simulink model "DP_STD_MDL_Boost"  (R2025a)
settings: Solver=VariableStepAuto  StartTime=0.0  StopTime=1  RelTol=1e-3
libraries: spsSeriesRLCBranchLib x4, peripheral_utilities x3, spsMosfetLib x2, spsControlledVoltageSourceLib x1, gmp_sil_core_pack x1, spsGroundLib x1, sps_lib x1
settings Model: SimulationMode=accelerator  Creator=javnson  LastModifiedBy=Lenovo

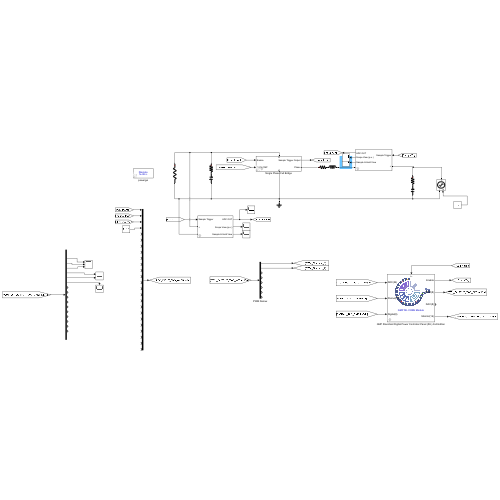
[thumbnail: Simulink's stored preview of the top-level diagram]
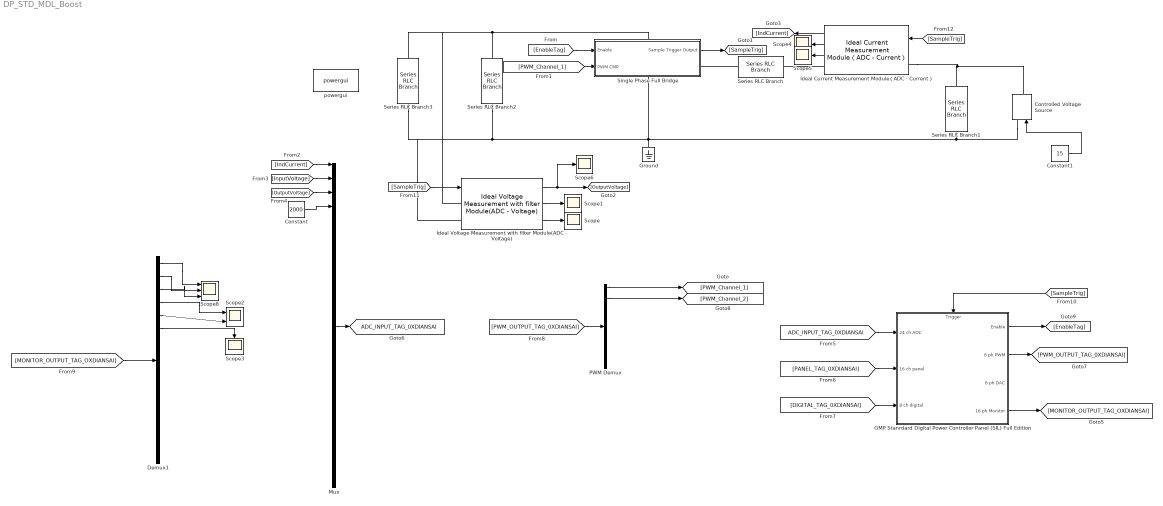
== system DP_STD_MDL_Boost ==
  Constant : Constant  Value=2000  OutDataTypeStr=uint32
  Constant1 : Constant  Value=15
  Controlled Voltage Source : spsControlledVoltageSourceLib/Controlled Voltage Source  Initialize=on  Source_Type=AC  Amplitude=0  Phase=0  Frequency=0  Measurements=None
  Demux1 : Demux  Outputs=16
  GMP Stanrdard Digital Power Controller Panel (SIL) Full Edition : Subsystem  mask(GMP SIL Core for single Motor Controller (full edition)){}
      mask help: This is GMP Motor Simulator port.
      settings: PortSchema="{\"entries\":[{\"content\":{\"sides\":[{\"content\":{\"connectorIds\":[\"In1\",\"In2\",\"In3\"]},\"type\":\"ConnectorPlacement.EquallySpacedRectSide\",\"uuid\":\"45c67bc9-9540-469a-a4ac-1e12eb9acca3\"},{\"content\":{\"connectorIds\":[\"Out1\",\"Out2\",\"Out3\",\"Out4\"],\"side\":\"RIGHT\"},\"type\":\"ConnectorPlacement.EquallySpacedRectSide\",\"uuid\":\"a17116b4-0460-48ab-8ada-a785da6c5e29\"},{\"content\":{\"connectorIds\":[\"In4\"],\"side\":\"TOP\"},\"type\":\"ConnectorPlacement.EquallySpacedRectSide\",\"uuid\":\"15623697-512e-4e4d-ab51-f53c2346fadb\"},{\"content\":{\"side\":\"BOTTOM\"},\"type\":\"ConnectorPlacement.EquallySpacedRectSide\",\"uuid\":\"47f7968c-22c1-4f3d-97d9-242e9dbf8d30\"}]},\"type\":\"ConnectorPlacement.EquallySpacedConnector\",\"uuid\":\"f369880c-e675-4c1f-982e-a4befb03f503\"}],\"packageUris\":[\"http://schema.mathworks.com/mf0/Connector/R2020b\"],\"version\":\"1.0\"}"
      mask DialogControl ParameterGroupVar Prompt: 参数
      mask Display:
      | image(append(fileparts(which('gmp_simulink_utilities.slx')),'\icon\GMP_Core.png'));
      | color('blue');
      | %text(0.3,0.3,'GMP SIL CORE Module','horizontalAlignment','left','verticalAlignment','bottom');
      | disp('\n\n\n\n\n\n\n\nGMP SIL CORE Module');
      | %text(0,0,'y=a*x^2+b','horizontalAlignment','middle', 'verticalAlignment','bottom');
      | 
      | 
      | module_pos = get_param(gcb, 'Position');
      | width = module_pos(3) - module_pos(1);
      | %rectangle('Position',[module_pos(1),module_pos(2),module_pos(3),module_pos(4)],'FaceColor','r');
      | 
      | color('Black');
      | 
      | port_label('output', 1, 'Enable');
      | port_label('output', 2, 'PWM(8)');
      | port_label('output', 3, 'DAC(8)');
      | port_label('output', 4, 'Monitor(16)');
      | 
      | port_label('input', 1, 'ADC(24)');
      | port_label('input', 2, 'Pannel(16)');
      | port_label('input', 3, 'Digital(8)');
      | port_label('input', 4, 'T');
  Ground : spsGroundLib/Ground  LConnTagsString=a
  Ideal Current Measurement Module（ADC - Current） : peripheral_utilities/Ideal Current Measurement Module（ADC - Current）  ADC_GAIN=0.005*20  ADC_BIT=12  ADC_REFERENCE=2.5  ADC_BIAS=0.9  ADC_INIT=0
      settings: SourceProductName=Virtual Peripheral Utilities
  Ideal Voltage Measurement with filter Module(ADC - Voltage) : peripheral_utilities/Ideal Voltage Measurement with filter Module(ADC - Voltage)  ADC_GAIN=0.0109  ADC_BIT=12  ADC_REFERENCE=2.5  ADC_BIAS=0.9966  ADC_INIT=0  cut_frequency=18e3
      settings: SourceProductName=Virtual Peripheral Utilities
  Mux : Mux  Inputs=24
  PWM Demux : Demux  Outputs=8
  Scope{,1,3..6} (6 alike) : Scope
      Scope settings: ActiveDisplayYMinimum=13.017568443143606  ActiveDisplayYMaximum=34.135422749659156  DataLoggingVariableName=ScopeData2
      Scope1 settings: ActiveDisplayYMinimum=0.36225  ActiveDisplayYMaximum=0.72612  DataLoggingVariableName=ScopeData3
      Scope3 settings: ActiveDisplayYMinimum=-0.10512  ActiveDisplayYMaximum=0.94605
      Scope4 settings: ActiveDisplayYMinimum=-0.05447  ActiveDisplayYMaximum=1.11716  DataLoggingVariableName=ScopeData4
      Scope5 settings: ActiveDisplayYMinimum=-12.976927448138717  ActiveDisplayYMaximum=22.918201693601077  DataLoggingVariableName=ScopeData5
      Scope6 settings: ActiveDisplayYMinimum=1322.762868000169  ActiveDisplayYMaximum=2949.7679787303091  DataLoggingVariableName=ScopeData7
  Scope2 : Scope  NumInputPorts=2
      settings: ActiveDisplayYMinimum=-1.03991  ActiveDisplayYMaximum=1.22666  DataLoggingVariableName=ScopeData3
  Scope8 : Scope  NumInputPorts=3
      settings: ActiveDisplayYMinimum=-1.4781145350127816  ActiveDisplayYMaximum=2.1253499910028788  DataLoggingVariableName=ScopeData9
  Series RLC Branch : spsSeriesRLCBranchLib/Series RLC Branch  LConnTagsString=__new0  RConnTagsString=__new0  BranchType=RL  Resistance=0.05  Inductance=680E-6  SetiL0=off  InitialCurrent=0  Capacitance=1e-6  Setx0=off  InitialVoltage=0  Measurements=None
  Series RLC Branch1 : spsSeriesRLCBranchLib/Series RLC Branch  LConnTagsString=__new0  RConnTagsString=__new0  BranchType=RC  Resistance=0.095  Inductance=1e-3  SetiL0=off  InitialCurrent=0  Capacitance=540E-6  Setx0=off  InitialVoltage=0  Measurements=None
  Series RLC Branch2 : spsSeriesRLCBranchLib/Series RLC Branch  LConnTagsString=__new0  RConnTagsString=__new0  BranchType=RC  Resistance=0.095  Inductance=1e-3  SetiL0=off  InitialCurrent=0  Capacitance=540E-6  Setx0=off  InitialVoltage=0  Measurements=None
  Series RLC Branch3 : spsSeriesRLCBranchLib/Series RLC Branch  LConnTagsString=__new0  RConnTagsString=__new0  BranchType=R  Resistance=30  Inductance=1e-3  SetiL0=off  InitialCurrent=0  Capacitance=1e-6  Setx0=off  InitialVoltage=0  Measurements=None
  Single Phase Full Bridge : Subsystem  AncestorBlock=peripheral_utilities/Single Phase Full Bridge  mask{fswitch=20e3, CMP_MAX=4200, Deadband_Upper=100, Deadband_Lower=100, Deadband_us=1.1905, phase_shift=0, R_mosfet_on=0.1, Lon=0, Rd=0.01, Vf=0.3, Rs=1e5, Cs=inf}
      mask init:
      | calculate_deadband(gcb, 'Deadband_Upper', 'Deadband_Lower',	'CMP_MAX', 'fswitch', 'Deadband_us');
      settings: PortSchema="{\"entries\":[{\"content\":{\"sides\":[{\"content\":{\"connectorIds\":[\"In1\",\"In2\"]},\"type\":\"ConnectorPlacement.EquallySpacedRectSide\",\"uuid\":\"20beeabc-b0ca-4337-b227-c7f02abd15d8\"},{\"content\":{\"connectorIds\":[\"Out1\",\"RConn1\"],\"side\":\"RIGHT\"},\"type\":\"ConnectorPlacement.EquallySpacedRectSide\",\"uuid\":\"a7923383-ac55-4621-ad1d-4d067c1fb84d\"},{\"content\":{\"connectorIds\":[\"LConn1\"],\"side\":\"TOP\"},\"type\":\"ConnectorPlacement.EquallySpacedRectSide\",\"uuid\":\"661bf0ae-1c96-4de8-96aa-28c06a0a56db\"},{\"content\":{\"connectorIds\":[\"RConn2\"],\"side\":\"BOTTOM\"},\"type\":\"ConnectorPlacement.EquallySpacedRectSide\",\"uuid\":\"fc2f6321-5787-4e1a-b5a2-65ed34db36b5\"}]},\"type\":\"ConnectorPlacement.EquallySpacedConnector\",\"uuid\":\"e2219b16-0a50-43ef-8183-c55a35d5a2a0\"}],\"packageUris\":[\"http://schema.mathworks.com/mf0/Connector/R2020b\"],\"version\":\"1.0\"}"
      mask Callback fswitch: calculate_deadband(gcb, 'Deadband_Upper', 'Deadband_Lower',	'CMP_MAX', 'fswitch', 'Deadband_us');
      mask Callback CMP_MAX: calculate_deadband(gcb, 'Deadband_Upper', 'Deadband_Lower',	'CMP_MAX', 'fswitch', 'Deadband_us');
      mask Callback Deadband_Upper: calculate_deadband(gcb, 'Deadband_Upper', 'Deadband_Lower',	'CMP_MAX', 'fswitch', 'Deadband_us');
      mask Callback Deadband_Lower: calculate_deadband(gcb, 'Deadband_Upper', 'Deadband_Lower',	'CMP_MAX', 'fswitch', 'Deadband_us');
      mask DialogControl DescGroupVar Prompt: Half Bridge With PWM Module
      mask DialogControl Control14 Prompt: GMP CTL Simulink Utilities: virtual peripherals
      mask DialogControl DescTextVar Prompt: This module provide a PWM (with deadband), and a MOSFET half bridge.
      mask DialogControl Container5 Prompt: PWM Modulator
      mask DialogControl ParameterGroupVar Prompt: PWM module parameters
      mask DialogControl Control2 Prompt: PWM Frequency (Hz):
      mask DialogControl Control3 Prompt: Full Scale PWM Compare value:
      mask DialogControl Control4 Prompt: (whole period is 2 * CMP_MAX ticks)
      mask DialogControl Control5 Prompt: Deadband Range Set (CMP Value):
      mask DialogControl Control6 Prompt: Single side deadband time: DEADBAND_CMP/2/CMP_MAX/fswitch
      mask DialogControl Control15 Prompt: Calculated Deadband, us
      mask DialogControl Control13 Prompt: Initial Phase Shift, unit rad
      mask DialogControl Container6 Prompt: MOSFET
      mask DialogControl Container3 Prompt: MOSFET parameters
      mask DialogControl Control7 Prompt: Rds(on), unit Ohm
      mask DialogControl Control8 Prompt: Internal diode inducctance, unit H
      mask DialogControl Control9 Prompt: Internal diode resistance Rd, unit Ohm
      mask DialogControl Control10 Prompt: Internal diode forward voltage Vf, unit V
      mask DialogControl Control11 Prompt: Snubber resistance Rs, unit ohm
      mask DialogControl Control12 Prompt: Snubber Capacitance Cs, unit F
  powergui : sps_lib/powergui  Priority=1  SimulationMode=Discrete  SampleTime=1e-6  frequency=60  Iterations=50  frequencyindice=0  Pbase=100e6  ErrMax=1e-4  UnitsV=kV  UnitsW=MW  buscounter=0  FunctionMessages=off  echomessages=off  EnableUseOfTLC=off  CurrentSourceSwitches=off  DisableSnubberDevices=off  DisableRonSwitches=off  DisableVfSwitches=off  DisplayEquations=off  AutomaticDiscreteSolvers=off  SolverType=Tustin/Backward Euler (TBE)  Interpol=off  ExternalGateDelay=off  methode=off  Ts=100  x0status=blocks  SPID=on  SwTol=0  HookPort=off  NonlinearTolerance=1e-4  nMaxIteration=100  ContinueOnMaxIteration=off  RestoreLinks=warning  ResistiveCurrentMeasurement=off  Frange=[0:2:500]  Ylog=off  Xlog=on  ShowGrid=off  save=off  variable=ZData  structure=0  ZoomFFT=off  StartTime=0.0  cycles=1  DisplayStyle=1  fundamental=60  FreqAxis=off  MaxFrequency=1000  frequencyindicesteady=1  RmsSteady=1  display=off
  tag scope: ADC_INPUT_TAG_0XDIANSAI=global
  wires:
  [SampleTrig] -> GMP Stanrdard Digital Power Controller Panel (SIL) Full Edition/4(Trigger)
  GMP Stanrdard Digital Power Controller Panel (SIL) Full Edition/1(Enable) -> [EnableTag]
  PWM Demux/1 -> [PWM_Channel_1]
  [IndCurrent] -> Mux/1
  [InputVoltage] -> Mux/2
  [OutputVoltage] -> Mux/3
  Mux/1 -> [ADC_INPUT_TAG_0XDIANSAI]
  [ADC_INPUT_TAG_0XDIANSAI] -> GMP Stanrdard Digital Power Controller Panel (SIL) Full Edition/1(24 ch ADC)
  [PANEL_TAG_0XDIANSAI] -> GMP Stanrdard Digital Power Controller Panel (SIL) Full Edition/2(16 ch panel)
  [DIGITAL_TAG_0XDIANSAI] -> GMP Stanrdard Digital Power Controller Panel (SIL) Full Edition/3(8 ch digital)
  [PWM_OUTPUT_TAG_0XDIANSAI] -> PWM Demux/1
  GMP Stanrdard Digital Power Controller Panel (SIL) Full Edition/2(8 ph PWM) -> [PWM_OUTPUT_TAG_0XDIANSAI]
  GMP Stanrdard Digital Power Controller Panel (SIL) Full Edition/4(16 ph Monitor) -> [MONITOR_OUTPUT_TAG_OXDIANSAI]
  [MONITOR_OUTPUT_TAG_OXDIANSAI] -> Demux1/1
  Demux1/4 -> Scope2/1
  Demux1/5 -> Scope2/2
  PWM Demux/2 -> [PWM_Channel_2]
  Demux1/6 -> Scope3/1
  Constant/1 -> Mux/4
  Constant1/1 -> Controlled Voltage Source/1
  [EnableTag] -> Single Phase Full Bridge/1(Enable)
  Single Phase Full Bridge/1(Sample Trigger Output) -> [SampleTrig]
  [PWM_Channel_1] -> Single Phase Full Bridge/2(PWM CMP)
  [SampleTrig] -> Ideal Voltage Measurement with filter Module(ADC - Voltage)/1
  Ideal Voltage Measurement with filter Module(ADC - Voltage)/1 -> Scope6/1, [OutputVoltage]
  Ideal Voltage Measurement with filter Module(ADC - Voltage)/3 -> Scope/1
  Ideal Voltage Measurement with filter Module(ADC - Voltage)/2 -> Scope1/1
  [SampleTrig] -> Ideal Current Measurement Module（ADC - Current）/1
  Ideal Current Measurement Module（ADC - Current）/1 -> [IndCurrent]
  Ideal Current Measurement Module（ADC - Current）/2 -> Scope4/1
  Ideal Current Measurement Module（ADC - Current）/3 -> Scope5/1
  Demux1/1 -> Scope8/1
  Demux1/2 -> Scope8/2
  Demux1/3 -> Scope8/3
  connections:
  Series RLC Branch/LConn1 -- Single Phase Full Bridge/RConn1
  Series RLC Branch1/LConn1 -- Ideal Current Measurement Module（ADC - Current）/LConn1 -- Controlled Voltage Source/RConn1
  Series RLC Branch2/LConn1 -- Ideal Voltage Measurement with filter Module(ADC - Voltage)/LConn1 -- Series RLC Branch3/LConn1 -- Single Phase Full Bridge/LConn1
  Controlled Voltage Source/LConn1 -- Ground/LConn1 -- Single Phase Full Bridge/RConn2 -- Ideal Voltage Measurement with filter Module(ADC - Voltage)/LConn2 -- Series RLC Branch3/RConn1 -- Series RLC Branch2/RConn1 -- Series RLC Branch1/RConn1
  Ideal Current Measurement Module（ADC - Current）/RConn1 -- Series RLC Branch/RConn1

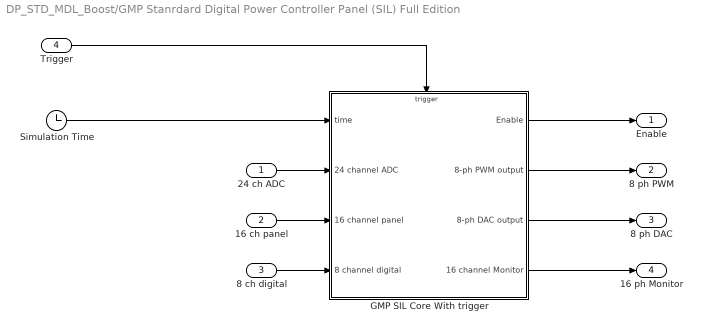
== system DP_STD_MDL_Boost/GMP Stanrdard Digital Power Controller Panel (SIL) Full Edition ==
  24 ch ADC : Inport
  16 ch panel : Inport  Port=2
  8 ch digital : Inport  Port=3
  Trigger : Inport  Port=4
  GMP SIL Core With trigger : Subsystem
  Simulation Time : Clock
  Enable : Outport
  8 ph PWM : Outport  Port=2
  8 ph DAC : Outport  Port=3
  16 ph Monitor : Outport  Port=4
  wires:
  GMP SIL Core With trigger/2(8-ph PWM output) -> 8 ph PWM/1
  Simulation Time/1 -> GMP SIL Core With trigger/1(time)
  GMP SIL Core With trigger/1(Enable) -> Enable/1
  16 ch panel/1 -> GMP SIL Core With trigger/3(16 channel panel)
  24 ch ADC/1 -> GMP SIL Core With trigger/2(24 channel ADC)
  GMP SIL Core With trigger/3(8-ph DAC output) -> 8 ph DAC/1
  Trigger/1 -> GMP SIL Core With trigger/Trigger
  8 ch digital/1 -> GMP SIL Core With trigger/4(8 channel digital)
  GMP SIL Core With trigger/4(16 channel Monitor) -> 16 ph Monitor/1

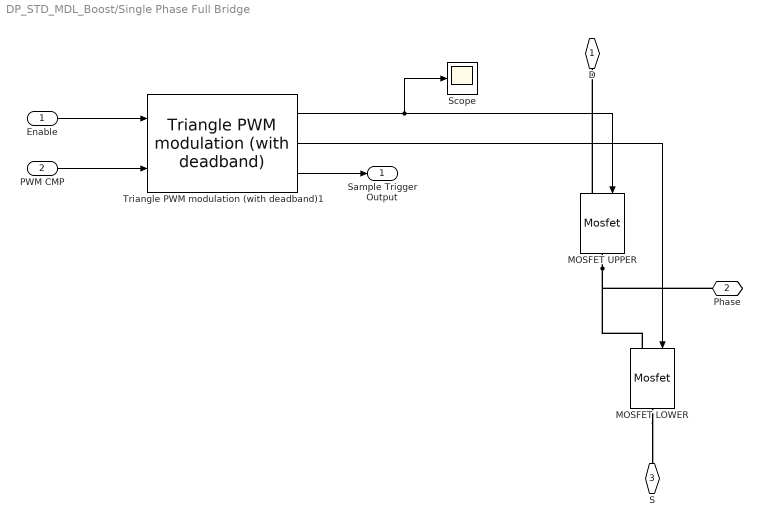
== system DP_STD_MDL_Boost/Single Phase Full Bridge ==
  Enable : Inport
  PWM CMP : Inport  Port=2
  MOSFET LOWER : spsMosfetLib/Mosfet  Ron=R_mosfet_on  Lon=Lon  Rd=Rd  Vfd=Vf  IC=0  Rs=Rs  Cs=Cs  Measurements=off
  MOSFET UPPER : spsMosfetLib/Mosfet  Ron=R_mosfet_on  Lon=Lon  Rd=Rd  Vfd=Vf  IC=0  Rs=Rs  Cs=Cs  Measurements=off
  Scope : Scope
      settings: DataLoggingVariableName=ScopeData6
  Triangle PWM modulation (with deadband)1 : peripheral_utilities/Triangle PWM modulation (with deadband)  fswitch=fswitch  CMP_MAX=CMP_MAX  Deadband_Upper=Deadband_Upper  Deadband_Lower=Deadband_Lower  phase_shift=phase_shift
      settings: SourceProductName=Virtual Peripheral Utilities
  D : PMIOPort  Side=Left
  Phase : PMIOPort  Port=2  Side=Right
  S : PMIOPort  Port=3  Side=Right
  Sample Trigger Output : Outport
  wires:
  PWM CMP/1 -> Triangle PWM modulation (with deadband)1/2
  Triangle PWM modulation (with deadband)1/2 -> MOSFET LOWER/1
  Triangle PWM modulation (with deadband)1/3 -> Sample Trigger Output/1
  Enable/1 -> Triangle PWM modulation (with deadband)1/1
  Triangle PWM modulation (with deadband)1/1 -> Scope/1, MOSFET UPPER/1
  connections:
  MOSFET LOWER/RConn1 -- S/RConn1
  MOSFET UPPER/RConn1 -- Phase/RConn1 -- MOSFET LOWER/LConn1
  MOSFET UPPER/LConn1 -- D/RConn1

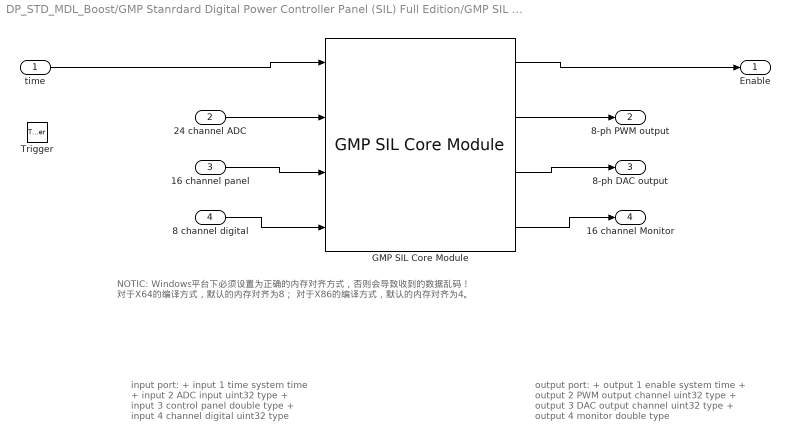
== system DP_STD_MDL_Boost/GMP Stanrdard Digital Power Controller Panel (SIL) Full Edition/GMP SIL Core With trigger ==
  note: input port:
      | + input 1 time system time
      | + input 2 ADC input uint32 type
      | + input 3 control panel double type
      | + input 4 channel digital uint32 type
  note: NOTIC:
      | Windows平台下必须设置为正确的内存对齐方式，否则会导致收到的数据乱码！
      | 对于X64的编译方式，默认的内存对齐为8；
      | 对于X86的编译方式，默认的内存对齐为4。
  note: output port:
      | + output 1 enable system time
      | + output 2 PWM output channel uint32 type
      | + output 3 DAC output channel uint32 type
      | + output 4 monitor double type
  time : Inport
  24 channel ADC : Inport  Port=2
  16 channel panel : Inport  Port=3
  8 channel digital : Inport  Port=4
  Trigger : TriggerPort  VariantControl=(inherit)  PortDimensions=1
  GMP SIL Core Module : gmp_sil_core_pack/GMP SIL Core Module  MaskPackedDataTypes={'double', 'uint32', 'double', 'int32'}  MaskPackedDataSizes={[1],[24],[16],[8]}  MaskUnpackedDataTypes={'double', 'uint32', 'uint32', 'double'}  MaskUnpackedDataSizes={[1],[8],[8],[16]}  MaskAlignment=1  MaskHostAddr='127.0.0.1'  MaskMsgTxPort=12500  MaskMsgRxPort=12501  MaskCmdTxPort=12502  MaskCmdRxPort=12503
      settings: SourceProductName=GMP SIL Core Utilities
  Enable : Outport
  8-ph PWM output : Outport  Port=2
  8-ph DAC output : Outport  Port=3
  16 channel Monitor : Outport  Port=4
  wires:
  24 channel ADC/1 -> GMP SIL Core Module/2
  16 channel panel/1 -> GMP SIL Core Module/3
  time/1 -> GMP SIL Core Module/1
  GMP SIL Core Module/3 -> 8-ph DAC output/1
  GMP SIL Core Module/2 -> 8-ph PWM output/1
  GMP SIL Core Module/1 -> Enable/1
  8 channel digital/1 -> GMP SIL Core Module/4
  GMP SIL Core Module/4 -> 16 channel Monitor/1
